simulink model "RearDifferentialController"  (R2026b)
undefined symbols (not defined in the file): PlntVehDstCGFrntAxl, PlntVehDstCGRearAxl
libraries: simulink x5, slpidlib x1, autolibutils x1
settings Model: Creator=The MathWorks, Inc.  LastModifiedBy=The MathWorks, Inc.

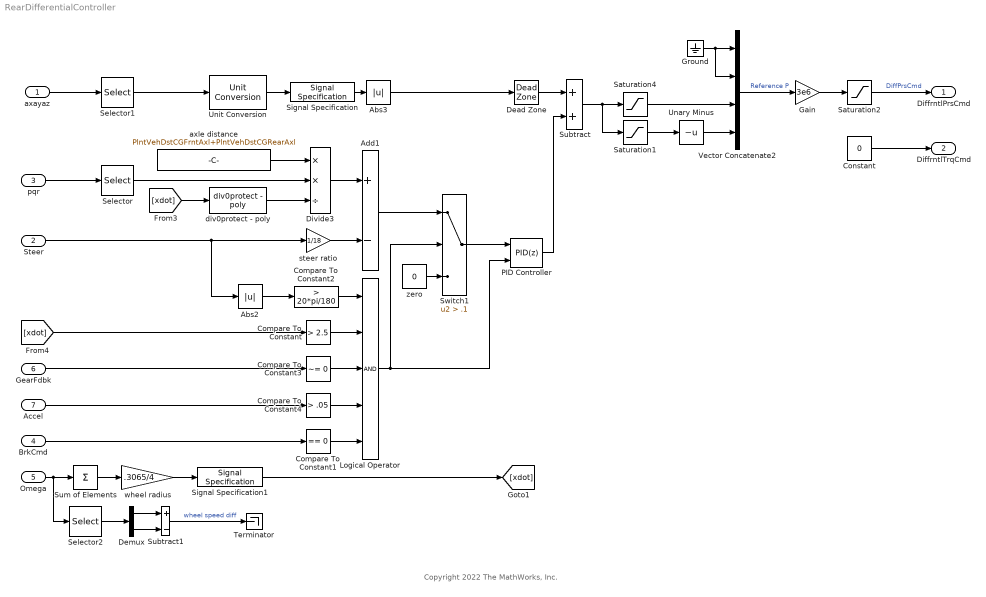
== system RearDifferentialController ==
  note: Copyright 2022 The MathWorks, Inc.
  axayaz : Inport  OutDataTypeStr=double  Unit=m/s^2  PortDimensions=3
  Steer : Inport  Port=2  OutDataTypeStr=double  PortDimensions=1
  pqr : Inport  Port=3  OutDataTypeStr=double  PortDimensions=3
  BrkCmd : Inport  Port=4  OutDataTypeStr=double  PortDimensions=1
  Omega : Inport  Port=5  OutDataTypeStr=double  Unit=rad/s  PortDimensions=4
  GearFdbk : Inport  Port=6  OutDataTypeStr=double  PortDimensions=1
  Accel : Inport  Port=7  OutDataTypeStr=double  PortDimensions=1
  Abs2 : Abs  SaturateOnIntegerOverflow=off
  Abs3 : Abs  ZeroCross=off  SaturateOnIntegerOverflow=off
  Add1 : Sum  Inputs=+-
  Compare To Constant : simulink/Logic and Bit Operations/Compare To Constant  relop=>  const=2.5  OutDataTypeStr=boolean
  Compare To Constant1 : simulink/Logic and Bit Operations/Compare To Constant  relop===  const=0  OutDataTypeStr=boolean
  Compare To Constant2 : simulink/Logic and Bit Operations/Compare To Constant  relop=>  const=20*pi/180  OutDataTypeStr=boolean
  Compare To Constant3 : simulink/Logic and Bit Operations/Compare To Constant  relop=~=  const=0  OutDataTypeStr=boolean
  Compare To Constant4 : simulink/Logic and Bit Operations/Compare To Constant  relop=>  const=.05  OutDataTypeStr=boolean
  Constant : Constant  Value=0  SampleTime=-1
  Dead Zone : DeadZone  ZeroCross=off
  Demux : Demux  Outputs=2
  Divide3 : Product  Inputs=**/
  Gain : Gain  Gain=3e6
  Ground : Ground
  Logical Operator : Logic  Inputs=5  AllPortsSameDT=off  OutDataTypeStr=boolean
  PID Controller : slpidlib/PID Controller  Controller=PID  Form=Parallel  TimeDomain=Discrete-time  UseExternalTs=off  SampleTime=-1  IntegratorMethod=Forward Euler  FilterMethod=Forward Euler  ControllerParametersSource=internal  P=1  I=.05  UseKiTs=off  D=0  UseExternalDerivativeSource=off  N=1  UseFilter=on  TunerSelectOption=Transfer Function Based (PID Tuner App)  ZeroCross=off  InitialConditionSource=internal  InitialConditionForIntegrator=0  InitialConditionForFilter=0  DifferentiatorICPrevScaledInput=0  ExternalReset=either  TrackingMode=off  Kt=1  LimitOutput=on  SatLimitsSource=internal  UpperSaturationLimit=1  LowerSaturationLimit=-1  LinearizeAsGain=on  AntiWindupMode=clamping  Kb=1  LimitIntegrator=off  UpperIntegratorSaturationLimit=inf  LowerIntegratorSaturationLimit=-inf  POutMin=[]  POutMax=[]  IOutMin=[]  IOutMax=[]  DOutMin=[]  DOutMax=[]  NOutMin=[]  NOutMax=[]  SumOutMin=[]  SumOutMax=[]  SaturationOutMin=[]  SaturationOutMax=[]  PParamMin=[]  PParamMax=[]  IParamMin=[]  IParamMax=[]  DParamMin=[]  DParamMax=[]  NParamMin=[]  NParamMax=[]  KbParamMin=[]  KbParamMax=[]  KtParamMin=[]  KtParamMax=[]  KbOutMin=[]  KbOutMax=[]  KtOutMin=[]  KtOutMax=[]  IntegratorOutMin=[]  IntegratorOutMax=[]  FilterOutMin=[]  FilterOutMax=[]  SumI1OutMin=[]  SumI1OutMax=[]  SumI2OutMin=[]  SumI2OutMax=[]  SumI3OutMin=[]  SumI3OutMax=[]  SumI4OutMin=[]  SumI4OutMax=[]  SumDOutMin=[]  SumDOutMax=[]  DifferentiatorOutMin=[]  DifferentiatorOutMax=[]  FilterDiffOutCoefMin=[]  FilterDiffOutCoefMax=[]  ReciprocalOutMin=[]  ReciprocalOutMax=[]  SumDenOutMin=[]  SumDenOutMax=[]  SumNumOutMin=[]  SumNumOutMax=[]  DivideOutMin=[]  DivideOutMax=[]  UdiffTsProdOutMin=[]  UdiffTsProdOutMax=[]  NTsProdOutMin=[]  NTsProdOutMax=[]  UintegralTsProdOutMin=[]  UintegralTsProdOutMax=[]  UngainTsProdOutMin=[]  UngainTsProdOutMax=[]  ClampingZeroOutDataTypeStr=Inherit: Inherit via back propagation  ClampingZeroOutMin=[]  ClampingZeroOutMax=[]  FilterDenConstantOutDataTypeStr=Inherit: Inherit via back propagation  FilterDenConstantOutMin=[]  FilterDenConstantOutMax=[]  PCopyOutDataTypeStr=Inherit: Inherit via back propagation  PCopyOutMin=[]  PCopyOutMax=[]  NCopyOutDataTypeStr=Inherit: Inherit via back propagation  NCopyOutMin=[]  NCopyOutMax=[]  IntegratorContinuousStateAttributes=''  IntegratorStateMustResolveToSignalObject=off  IntegratorRTWStateStorageClass=Auto  FilterContinuousStateAttributes=''  FilterStateMustResolveToSignalObject=off  FilterRTWStateStorageClass=Auto  ParallelPVariant=InternalParameters  IdealPVariant=Disabled  IVariant=InternalParameters  DVariant=InternalParameters  IntegratorVariant=Discrete  SatVariant=Enabled  AWVariant=DiscClampingParallel  PCopyVariant=Disabled  TRVariant=Disabled  FdbkBlocksVariant=Forward  IdealPFdbkVariant=Disabled  SatFdbkVariant=Disabled  DerivativeFilterVariant=ForwardEulerFilter  NVariant=InternalParameters  NCopyVariant=Disabled  FilterICVariant=InternalICsFilter  IntegratorICVariant=InternalICs  ExternalResetVariant=ExternalReset  TRSumVariant=Passthrough  SumFdbkVariant=Disabled  SumVariant=Sum_PID  TsampFilterVariant=InternalTs  TsampNgainVariant=Passthrough  TsampIntegralVariant=Disabled_SignalSpec  ExternalSaturationOutDataTypeStr=Inherit: Same as second input  DerivativeSourceVariant=ErrorSignal  PreIntVariant=InternalPreInt
  Saturation1 : Saturate  UpperLimit=0  LowerLimit=-1  ZeroCross=off
  Saturation2 : Saturate  UpperLimit=5e6  LowerLimit=0  ZeroCross=off
  Saturation4 : Saturate  UpperLimit=1  LowerLimit=0  ZeroCross=off
  Selector : Selector  InputPortWidth=3  IndexOptions=Index vector (dialog)  Indices=[3]  OutputSizes=1  RuntimeRangeChecks=off
  Selector1 : Selector  InputPortWidth=3  IndexOptions=Index vector (dialog)  Indices=[2]  OutputSizes=1  RuntimeRangeChecks=off
  Selector2 : Selector  InputPortWidth=4  IndexOptions=Index vector (dialog)  Indices=[3 4]  OutputSizes=1  RuntimeRangeChecks=off
  Signal Specification : SignalSpecification  Unit=gn
  Signal Specification1 : SignalSpecification  Unit=m/s
  Subtract : Sum
  Subtract1 : Sum  Inputs=+-
  Sum of Elements : Sum  Inputs=+
  Switch1 : Switch  Criteria=u2 > Threshold  Threshold=.1  SaturateOnIntegerOverflow=off  InputSameDT=off
  Terminator : Terminator
  Unary Minus : UnaryMinus
  Unit Conversion : UnitConversion
  Vector Concatenate2 : Concatenate  NumInputs=4
  axle distance : Constant  Value=PlntVehDstCGFrntAxl+PlntVehDstCGRearAxl
  div0protect - poly : autolibutils/div0protect - poly  thresh=1  ZeroCross1=on  aMode=6
  steer ratio : Gain  Gain=1/18
  wheel radius : Gain  Gain=.3065/4
  zero : Constant  Value=0
  DiffrntlPrsCmd : Outport  OutDataTypeStr=double  PortDimensions=4  VectorParamsAs1DForOutWhenUnconnected=off
  DiffrntlTrqCmd : Outport  Port=2  OutDataTypeStr=double  PortDimensions=1  VectorParamsAs1DForOutWhenUnconnected=off
  wires:
  Compare To Constant4/1 -> Logical Operator/4
  Signal Specification1/1 -> [xdot]
  div0protect - poly/1 -> Divide3/3
  Abs2/1 -> Compare To Constant2/1
  steer ratio/1 -> Add1/2
  axayaz/1 -> Selector1/1
  Subtract1/1 -> Terminator/1  "wheel speed diff"
  Selector2/1 -> Demux/1
  Selector1/1 -> Unit Conversion/1
  Add1/1 -> Switch1/1
  Saturation2/1 -> DiffrntlPrsCmd/1  "DiffPrsCmd"
  Demux/1 -> Subtract1/1
  Constant/1 -> DiffrntlTrqCmd/1
  PID Controller/1 -> Subtract/2
  Divide3/1 -> Add1/1
  GearFdbk/1 -> Compare To Constant3/1
  Subtract/1 -> Saturation1/1, Saturation4/1
  Compare To Constant3/1 -> Logical Operator/3
  Logical Operator/1 -> PID Controller/2, Switch1/2
  Signal Specification/1 -> Abs3/1
  Accel/1 -> Compare To Constant4/1
  Abs3/1 -> Dead Zone/1
  Sum of Elements/1 -> wheel radius/1
  wheel radius/1 -> Signal Specification1/1
  Steer/1 -> Abs2/1, steer ratio/1
  Unary Minus/1 -> Vector Concatenate2/4
  Compare To Constant2/1 -> Logical Operator/1
  Compare To Constant/1 -> Logical Operator/2
  Switch1/1 -> PID Controller/1
  Omega/1 -> Selector2/1, Sum of Elements/1
  Dead Zone/1 -> Subtract/1
  [xdot] -> Compare To Constant/1
  BrkCmd/1 -> Compare To Constant1/1
  Selector/1 -> Divide3/2
  Demux/2 -> Subtract1/2
  Ground/1 -> Vector Concatenate2/2, Vector Concatenate2/1
  Compare To Constant1/1 -> Logical Operator/5
  pqr/1 -> Selector/1
  Unit Conversion/1 -> Signal Specification/1
  Gain/1 -> Saturation2/1
  Saturation1/1 -> Unary Minus/1
  zero/1 -> Switch1/3
  Vector Concatenate2/1 -> Gain/1  "Reference P"
  [xdot] -> div0protect - poly/1
  axle distance/1 -> Divide3/1
  Saturation4/1 -> Vector Concatenate2/3
